simulink library "MFMdl6"  (Simulink 8.8)
settings: Solver=VariableStepAuto  StartTime=0.0  StopTime=10.0  RelTol=1e-3
libraries: simulink x4
settings Model: Creator=viett  LastModifiedBy=viett

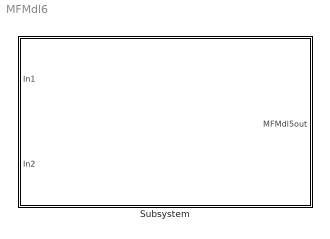
== system MFMdl6 ==
  Subsystem : Subsystem

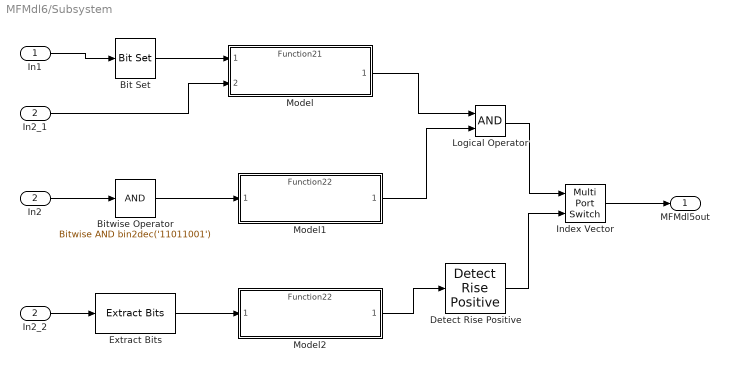
== system MFMdl6/Subsystem ==
  In1 : Inport
  In2 : Inport  Port=2
  Bit Set : simulink/Logic and Bit Operations/Bit Set  iBit=0
  Bitwise Operator : simulink/Logic and Bit Operations/Bitwise Operator  logicop=AND  UseBitMask=on  BitMask=bin2dec('11011001')  BitMaskRealWorld=Stored Integer
  Detect Rise Positive : simulink/Logic and Bit Operations/Detect Rise Positive  vinit=0  OutDataTypeStr=boolean
  Extract Bits : simulink/Logic and Bit Operations/Extract Bits  bitsToExtract=Upper half  numBits=8  bitIdxRange=[0 7]  outScalingMode=Preserve fixed-point scaling
  In2_1 : InportShadow  Port=2
  In2_2 : InportShadow  Port=2
  Index Vector : MultiPortSwitch  DataPortOrder=Zero-based contiguous  Inputs=1  zeroidx=on
  Logical Operator : Logic  AllPortsSameDT=off  OutDataTypeStr=boolean
  Model : ModelReference  ModelNameDialog=Function21.slx  SimulationMode=Normal  ModelReferenceVersion=1.3
  Model1 : ModelReference  ModelNameDialog=Function22.slx  SimulationMode=Normal  ModelReferenceVersion=1.3
  Model2 : ModelReference  ModelNameDialog=Function22.slx  SimulationMode=Normal  ModelReferenceVersion=1.3
  MFMdl5out : Outport
  wires:
  In1/1 -> Bit Set/1
  In2_2/1 -> Extract Bits/1
  Detect Rise Positive/1 -> Index Vector/2
  Bitwise Operator/1 -> Model1/1
  Model/1 -> Logical Operator/1
  Model1/1 -> Logical Operator/2
  Bit Set/1 -> Model/1
  Model2/1 -> Detect Rise Positive/1
  Extract Bits/1 -> Model2/1
  Logical Operator/1 -> Index Vector/1
  Index Vector/1 -> MFMdl5out/1
  In2_1/1 -> Model/2
  In2/1 -> Bitwise Operator/1
